simulink library "rewardLibrary"  (R2022b)
settings: Solver=VariableStepAuto  StartTime=0.0  StopTime=10.0  RelTol=1e-3
values from neighbouring files (symbols this model uses):
  accel_vec = (-4:0.5:4)'    [setUpModel.m]
  Ts = 0.1    [setUpMPC.m]
  TsRL = Ts    [setUpRLEnv.m]
  vel_vec = 0:2:20    [setUpModel.m]
undefined symbols (not defined in the file or in its folder): A, B, C, curvature1, D, D_default, DiscIntNeverNeededParam, E, F, gradbp1, k_sigmoid, steer_lim, t_gap, v_set, x_colpen, y_colpen, Z_colpen
libraries: simulink x379, $bdroot x2, mpcadaslib x1
(part 3 of 9)

== system rewardLibrary/Obs // Reward 8-9 ==
  xgap : Inport
  ygap : Inport  Port=2
  v_lead : Inport  Port=3
  v_ego : Inport  Port=4
  v_ref : Inport  Port=5
  e1 : Inport  Port=6
  e2 : Inport  Port=7
  e1dot : Inport  Port=8
  e2dot : Inport  Port=9
  accel : Inport  Port=10
  steer : Inport  Port=11
  collided : Inport  Port=12
  A : Gain  Gain=0
  Abs : Abs  SaturateOnIntegerOverflow=off
  B : Gain  Gain=2000
  Compare To Constant : simulink/Logic and Bit Operations/Compare To Constant  relop=<=  const=6  OutDataTypeStr=boolean
  E : Gain  Gain=2000
  Gain1 : Gain  Gain=20
  Logical Operator1 : Logic  Operator=OR  Inputs=3  AllPortsSameDT=off  OutDataTypeStr=boolean
  Overtaking : Subsystem
  Path following : Subsystem
  Subsystem : Subsystem
  Subsystem2 : Subsystem
  Sum : Sum  Inputs=--+++++
  Zone collision penalty : Lookup_n-D  BreakpointsForDimension1=y_colpen  BreakpointsForDimension2=x_colpen  Table=Z_colpen  ExtrapMethod=Clip  InternalRulePriority=Speed  RndMeth=Simplest
      settings: InputPortMap=u0,u1
      mask Display:
      | image("LookupTable.PNG")
      | port_label('input', 1, 'y')
      | port_label('input', 2, 'x')
      | port_label('output', 1, 'p_col')
  obs : Outport  VectorParamsAs1DForOutWhenUnconnected=off
  Reward : Outport  Port=2  VectorParamsAs1DForOutWhenUnconnected=off
  isDone : Outport  Port=3  VectorParamsAs1DForOutWhenUnconnected=off
  tag scope: onTrack=global, p_col=global
  wires:
  Zone collision penalty/1 -> [p_col], Sum/7
  E/1 -> Sum/2
  Subsystem2/2(failCollided) -> Logical Operator1/2, E/1
  Overtaking/1(r_ot) -> Sum/6
  B/1 -> Sum/4
  Subsystem2/4(overtakeSuccess) -> B/1
  [ry2] -> Overtaking/1(ry)
  Path following/1(r_pf) -> Sum/5
  e2dot/1 -> Subsystem/6(e2dot)
  e1/1 -> Abs/1, Path following/2(e1), Subsystem/3(e1), Subsystem2/2(e1)
  e2/1 -> Subsystem/4(e2), Path following/3(e2), Subsystem2/3(e2)
  v_lead/1 -> Subsystem/7(v_lead)
  xgap/1 -> Subsystem/8(xgap), Subsystem2/4(xgap), Zone collision penalty/2, Overtaking/2(G)
  Subsystem/1(obs) -> obs/1
  e1dot/1 -> Subsystem/5(e1dot)
  Sum/1 -> Reward/1
  Gain1/1 -> Sum/1
  Abs/1 -> Compare To Constant/1
  Compare To Constant/1 -> [onTrack]
  collided/1 -> Subsystem2/5(collided)
  v_ref/1 -> Subsystem/2(v_ref)
  ygap/1 -> Subsystem/9(ygap), Zone collision penalty/1
  Subsystem/2(v_err) -> Path following/1(v_err)
  steer/1 -> Path following/4(steer)
  accel/1 -> Path following/5(accel)
  Logical Operator1/1 -> isDone/1
  v_ego/1 -> Subsystem2/1(v_ego), Subsystem/1(v_ego)
  Subsystem2/1(fail) -> Logical Operator1/1, Gain1/1
  Subsystem2/3(completeCourse) -> A/1, Logical Operator1/3
  A/1 -> Sum/3

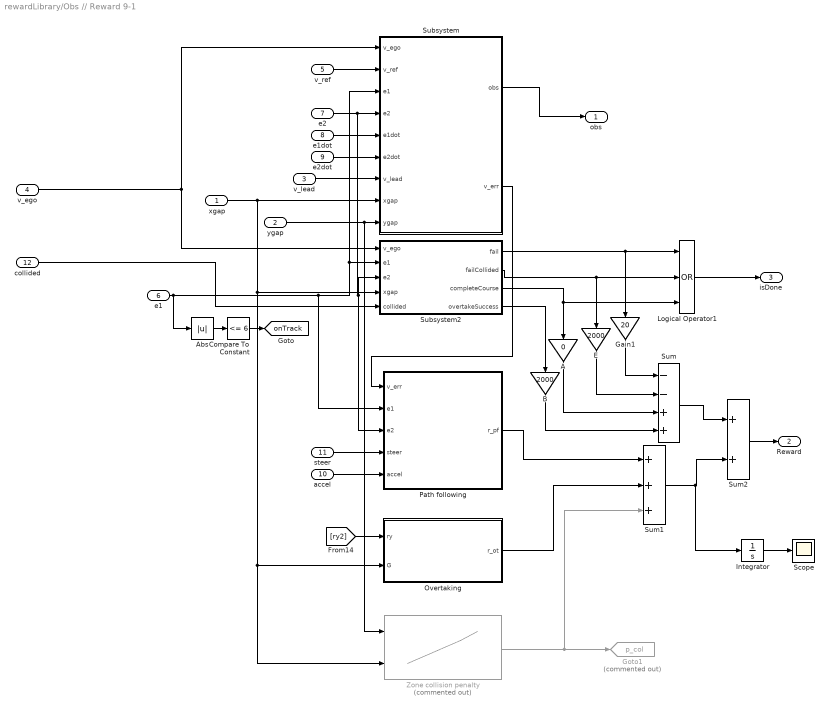
== system rewardLibrary/Obs // Reward 9-1 ==
  xgap : Inport
  ygap : Inport  Port=2
  v_lead : Inport  Port=3
  v_ego : Inport  Port=4
  v_ref : Inport  Port=5
  e1 : Inport  Port=6
  e2 : Inport  Port=7
  e1dot : Inport  Port=8
  e2dot : Inport  Port=9
  accel : Inport  Port=10
  steer : Inport  Port=11
  collided : Inport  Port=12
  A : Gain  Gain=0
  Abs : Abs  SaturateOnIntegerOverflow=off
  B : Gain  Gain=2000
  Compare To Constant : simulink/Logic and Bit Operations/Compare To Constant  relop=<=  const=6  OutDataTypeStr=boolean
  E : Gain  Gain=2000
  Gain1 : Gain  Gain=20
  Goto1 : Goto  Commented=on  GotoTag=p_col  TagVisibility=global
  Integrator : Integrator
  Logical Operator1 : Logic  Operator=OR  Inputs=3  AllPortsSameDT=off  OutDataTypeStr=boolean
  Overtaking : Subsystem
  Path following : Subsystem
  Scope : Scope
  Subsystem : Subsystem
  Subsystem2 : Subsystem
  Sum : Sum  Inputs=--++
  Sum1 : Sum  Inputs=+++
  Sum2 : Sum
  Zone collision penalty : Lookup_n-D  Commented=on  BreakpointsForDimension1=y_colpen  BreakpointsForDimension2=x_colpen  Table=Z_colpen  ExtrapMethod=Clip  InternalRulePriority=Speed  RndMeth=Simplest
      settings: InputPortMap=u0,u1
      mask Display:
      | image("LookupTable.PNG")
      | port_label('input', 1, 'y')
      | port_label('input', 2, 'x')
      | port_label('output', 1, 'p_col')
  obs : Outport  VectorParamsAs1DForOutWhenUnconnected=off
  Reward : Outport  Port=2  VectorParamsAs1DForOutWhenUnconnected=off
  isDone : Outport  Port=3  VectorParamsAs1DForOutWhenUnconnected=off
  tag scope: onTrack=global
  wires:
  Zone collision penalty/1 -> Sum1/3, Goto1/1
  E/1 -> Sum/2
  Subsystem2/2(failCollided) -> Logical Operator1/2, E/1
  Overtaking/1(r_ot) -> Sum1/2
  B/1 -> Sum/4
  Subsystem2/4(overtakeSuccess) -> B/1
  [ry2] -> Overtaking/1(ry)
  Path following/1(r_pf) -> Sum1/1
  e2dot/1 -> Subsystem/6(e2dot)
  e1/1 -> Abs/1, Path following/2(e1), Subsystem/3(e1), Subsystem2/2(e1)
  e2/1 -> Subsystem/4(e2), Path following/3(e2), Subsystem2/3(e2)
  v_lead/1 -> Subsystem/7(v_lead)
  xgap/1 -> Subsystem/8(xgap), Subsystem2/4(xgap), Zone collision penalty/2, Overtaking/2(G)
  Subsystem/1(obs) -> obs/1
  e1dot/1 -> Subsystem/5(e1dot)
  Gain1/1 -> Sum/1
  Abs/1 -> Compare To Constant/1
  Compare To Constant/1 -> [onTrack]
  collided/1 -> Subsystem2/5(collided)
  v_ref/1 -> Subsystem/2(v_ref)
  ygap/1 -> Subsystem/9(ygap), Zone collision penalty/1
  Subsystem/2(v_err) -> Path following/1(v_err)
  steer/1 -> Path following/4(steer)
  accel/1 -> Path following/5(accel)
  Logical Operator1/1 -> isDone/1
  v_ego/1 -> Subsystem2/1(v_ego), Subsystem/1(v_ego)
  Subsystem2/1(fail) -> Logical Operator1/1, Gain1/1
  Subsystem2/3(completeCourse) -> A/1, Logical Operator1/3
  A/1 -> Sum/3
  Sum2/1 -> Reward/1
  Sum/1 -> Sum2/1
  Sum1/1 -> Integrator/1, Sum2/2
  Integrator/1 -> Scope/1

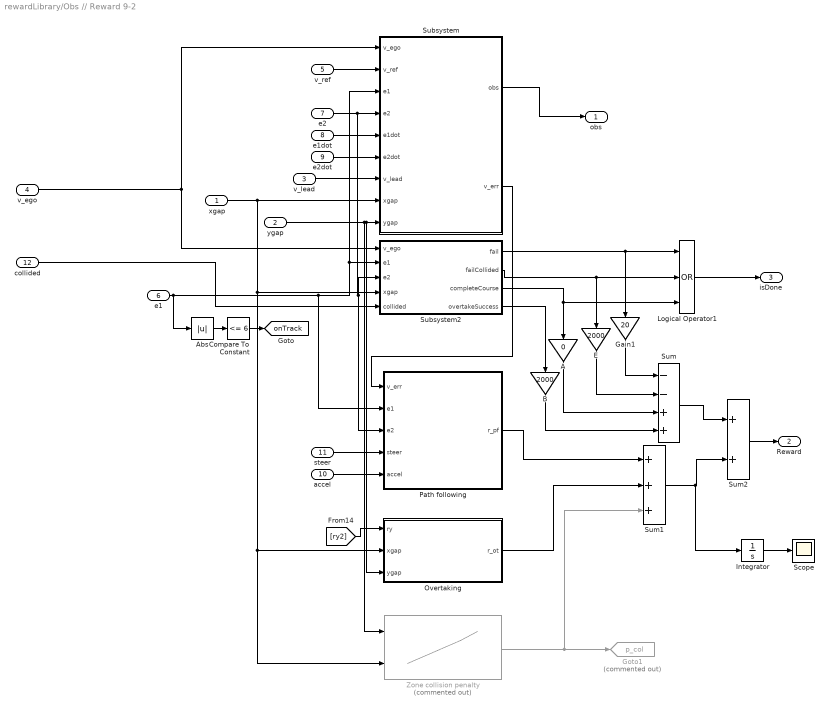
== system rewardLibrary/Obs // Reward 9-2 ==
  xgap : Inport
  ygap : Inport  Port=2
  v_lead : Inport  Port=3
  v_ego : Inport  Port=4
  v_ref : Inport  Port=5
  e1 : Inport  Port=6
  e2 : Inport  Port=7
  e1dot : Inport  Port=8
  e2dot : Inport  Port=9
  accel : Inport  Port=10
  steer : Inport  Port=11
  collided : Inport  Port=12
  A : Gain  Gain=0
  Abs : Abs  SaturateOnIntegerOverflow=off
  B : Gain  Gain=2000
  Compare To Constant : simulink/Logic and Bit Operations/Compare To Constant  relop=<=  const=6  OutDataTypeStr=boolean
  E : Gain  Gain=2000
  Gain1 : Gain  Gain=20
  Goto1 : Goto  Commented=on  GotoTag=p_col  TagVisibility=global
  Integrator : Integrator
  Logical Operator1 : Logic  Operator=OR  Inputs=3  AllPortsSameDT=off  OutDataTypeStr=boolean
  Overtaking : Subsystem
  Path following : Subsystem
  Scope : Scope
  Subsystem : Subsystem
  Subsystem2 : Subsystem
  Sum : Sum  Inputs=--++
  Sum1 : Sum  Inputs=+++
  Sum2 : Sum
  Zone collision penalty : Lookup_n-D  Commented=on  BreakpointsForDimension1=y_colpen  BreakpointsForDimension2=x_colpen  Table=Z_colpen  ExtrapMethod=Clip  InternalRulePriority=Speed  RndMeth=Simplest
      settings: InputPortMap=u0,u1
      mask Display:
      | image("LookupTable.PNG")
      | port_label('input', 1, 'y')
      | port_label('input', 2, 'x')
      | port_label('output', 1, 'p_col')
  obs : Outport  VectorParamsAs1DForOutWhenUnconnected=off
  Reward : Outport  Port=2  VectorParamsAs1DForOutWhenUnconnected=off
  isDone : Outport  Port=3  VectorParamsAs1DForOutWhenUnconnected=off
  tag scope: onTrack=global
  wires:
  Zone collision penalty/1 -> Sum1/3, Goto1/1
  E/1 -> Sum/2
  Subsystem2/2(failCollided) -> Logical Operator1/2, E/1
  Overtaking/1(r_ot) -> Sum1/2
  B/1 -> Sum/4
  Subsystem2/4(overtakeSuccess) -> B/1
  [ry2] -> Overtaking/1(ry)
  Path following/1(r_pf) -> Sum1/1
  e2dot/1 -> Subsystem/6(e2dot)
  e1/1 -> Abs/1, Path following/2(e1), Subsystem/3(e1), Subsystem2/2(e1)
  e2/1 -> Subsystem/4(e2), Path following/3(e2), Subsystem2/3(e2)
  v_lead/1 -> Subsystem/7(v_lead)
  xgap/1 -> Subsystem/8(xgap), Subsystem2/4(xgap), Zone collision penalty/2, Overtaking/2(xgap)
  Subsystem/1(obs) -> obs/1
  e1dot/1 -> Subsystem/5(e1dot)
  Gain1/1 -> Sum/1
  Abs/1 -> Compare To Constant/1
  Compare To Constant/1 -> [onTrack]
  collided/1 -> Subsystem2/5(collided)
  v_ref/1 -> Subsystem/2(v_ref)
  ygap/1 -> Overtaking/3(ygap), Subsystem/9(ygap), Zone collision penalty/1
  Subsystem/2(v_err) -> Path following/1(v_err)
  steer/1 -> Path following/4(steer)
  accel/1 -> Path following/5(accel)
  Logical Operator1/1 -> isDone/1
  v_ego/1 -> Subsystem2/1(v_ego), Subsystem/1(v_ego)
  Subsystem2/1(fail) -> Logical Operator1/1, Gain1/1
  Subsystem2/3(completeCourse) -> A/1, Logical Operator1/3
  A/1 -> Sum/3
  Sum2/1 -> Reward/1
  Sum/1 -> Sum2/1
  Sum1/1 -> Integrator/1, Sum2/2
  Integrator/1 -> Scope/1

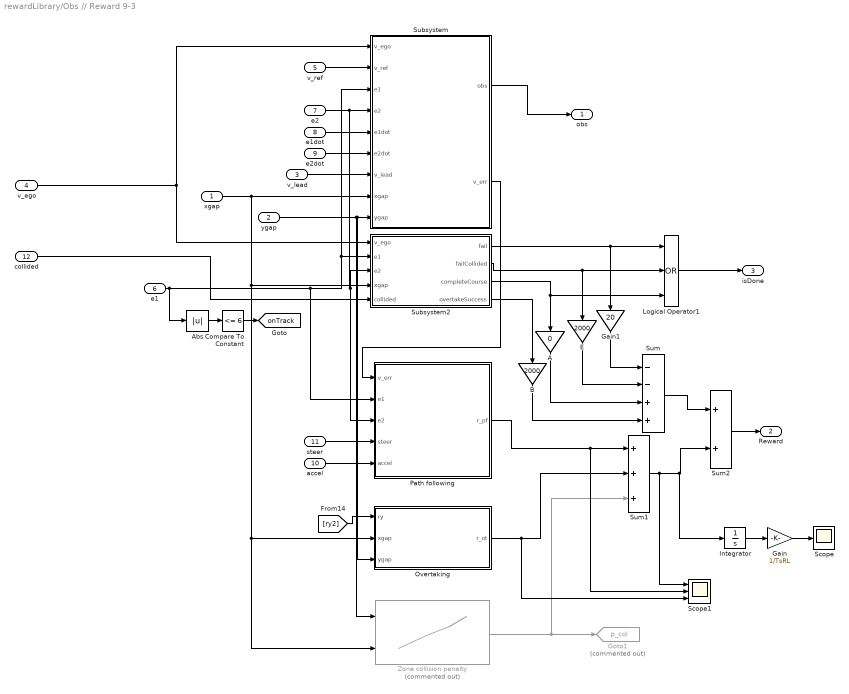
== system rewardLibrary/Obs // Reward 9-3 ==
  xgap : Inport
  ygap : Inport  Port=2
  v_lead : Inport  Port=3
  v_ego : Inport  Port=4
  v_ref : Inport  Port=5
  e1 : Inport  Port=6
  e2 : Inport  Port=7
  e1dot : Inport  Port=8
  e2dot : Inport  Port=9
  accel : Inport  Port=10
  steer : Inport  Port=11
  collided : Inport  Port=12
  A : Gain  Gain=0
  Abs : Abs  SaturateOnIntegerOverflow=off
  B : Gain  Gain=2000
  Compare To Constant : simulink/Logic and Bit Operations/Compare To Constant  relop=<=  const=6  OutDataTypeStr=boolean
  E : Gain  Gain=2000
  Gain : Gain  Gain=1/TsRL
  Gain1 : Gain  Gain=20
  Goto1 : Goto  Commented=on  GotoTag=p_col  TagVisibility=global
  Integrator : Integrator
  Logical Operator1 : Logic  Operator=OR  Inputs=3  AllPortsSameDT=off  OutDataTypeStr=boolean
  Overtaking : Subsystem
  Path following : Subsystem
  Scope : Scope
  Scope1 : Scope  NumInputPorts=3
  Subsystem : Subsystem
  Subsystem2 : Subsystem
  Sum : Sum  Inputs=--++
  Sum1 : Sum  Inputs=+++
  Sum2 : Sum
  Zone collision penalty : Lookup_n-D  Commented=on  BreakpointsForDimension1=y_colpen  BreakpointsForDimension2=x_colpen  Table=Z_colpen  ExtrapMethod=Clip  InternalRulePriority=Speed  RndMeth=Simplest
      settings: InputPortMap=u0,u1
      mask Display:
      | image("LookupTable.PNG")
      | port_label('input', 1, 'y')
      | port_label('input', 2, 'x')
      | port_label('output', 1, 'p_col')
  obs : Outport  VectorParamsAs1DForOutWhenUnconnected=off
  Reward : Outport  Port=2  VectorParamsAs1DForOutWhenUnconnected=off
  isDone : Outport  Port=3  VectorParamsAs1DForOutWhenUnconnected=off
  tag scope: onTrack=global
  wires:
  Zone collision penalty/1 -> Sum1/3, Goto1/1
  E/1 -> Sum/2
  Subsystem2/2(failCollided) -> Logical Operator1/2, E/1
  Overtaking/1(r_ot) -> Scope1/3, Sum1/2
  B/1 -> Sum/4
  Subsystem2/4(overtakeSuccess) -> B/1
  [ry2] -> Overtaking/1(ry)
  Path following/1(r_pf) -> Scope1/2, Sum1/1
  e2dot/1 -> Subsystem/6(e2dot)
  e1/1 -> Abs/1, Path following/2(e1), Subsystem/3(e1), Subsystem2/2(e1)
  e2/1 -> Subsystem/4(e2), Path following/3(e2), Subsystem2/3(e2)
  v_lead/1 -> Subsystem/7(v_lead)
  xgap/1 -> Subsystem/8(xgap), Subsystem2/4(xgap), Zone collision penalty/2, Overtaking/2(xgap)
  Subsystem/1(obs) -> obs/1
  e1dot/1 -> Subsystem/5(e1dot)
  Gain1/1 -> Sum/1
  Abs/1 -> Compare To Constant/1
  Compare To Constant/1 -> [onTrack]
  collided/1 -> Subsystem2/5(collided)
  v_ref/1 -> Subsystem/2(v_ref)
  ygap/1 -> Overtaking/3(ygap), Subsystem/9(ygap), Zone collision penalty/1
  Subsystem/2(v_err) -> Path following/1(v_err)
  steer/1 -> Path following/4(steer)
  accel/1 -> Path following/5(accel)
  Logical Operator1/1 -> isDone/1
  v_ego/1 -> Subsystem2/1(v_ego), Subsystem/1(v_ego)
  Subsystem2/1(fail) -> Logical Operator1/1, Gain1/1
  Subsystem2/3(completeCourse) -> A/1, Logical Operator1/3
  A/1 -> Sum/3
  Sum2/1 -> Reward/1
  Sum/1 -> Sum2/1
  Sum1/1 -> Scope1/1, Integrator/1, Sum2/2
  Gain/1 -> Scope/1
  Integrator/1 -> Gain/1

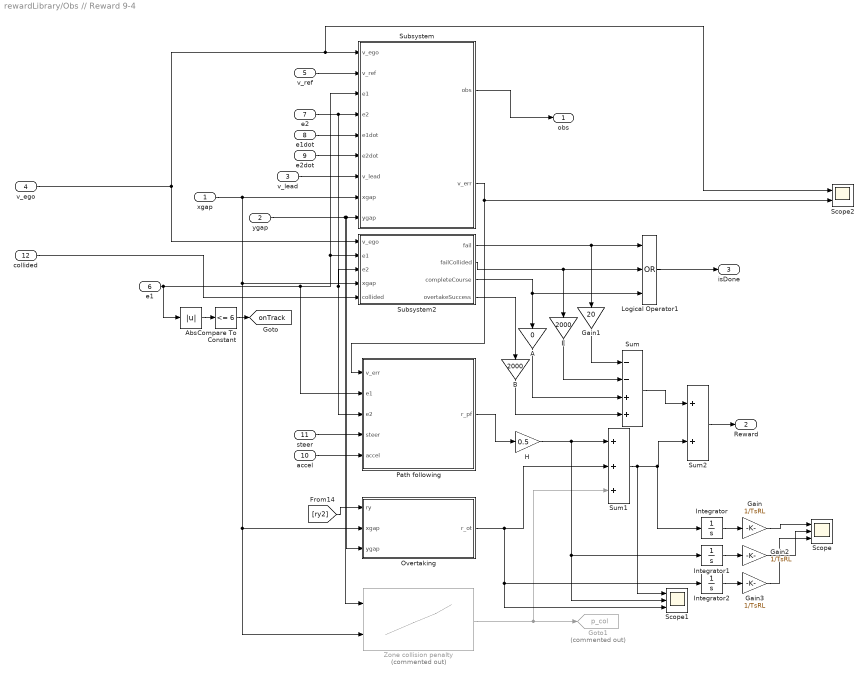
== system rewardLibrary/Obs // Reward 9-4 ==
  xgap : Inport
  ygap : Inport  Port=2
  v_lead : Inport  Port=3
  v_ego : Inport  Port=4
  v_ref : Inport  Port=5
  e1 : Inport  Port=6
  e2 : Inport  Port=7
  e1dot : Inport  Port=8
  e2dot : Inport  Port=9
  accel : Inport  Port=10
  steer : Inport  Port=11
  collided : Inport  Port=12
  A : Gain  Gain=0
  Abs : Abs  SaturateOnIntegerOverflow=off
  B : Gain  Gain=2000
  Compare To Constant : simulink/Logic and Bit Operations/Compare To Constant  relop=<=  const=6  OutDataTypeStr=boolean
  E : Gain  Gain=2000
  Gain : Gain  Gain=1/TsRL
  Gain1 : Gain  Gain=20
  Gain2 : Gain  Gain=1/TsRL
  Gain3 : Gain  Gain=1/TsRL
  Goto1 : Goto  Commented=on  GotoTag=p_col  TagVisibility=global
  H : Gain  Gain=0.5
  Integrator : Integrator
  Integrator1 : Integrator
  Integrator2 : Integrator
  Logical Operator1 : Logic  Operator=OR  Inputs=3  AllPortsSameDT=off  OutDataTypeStr=boolean
  Overtaking : Subsystem
  Path following : Subsystem
  Scope : Scope  NumInputPorts=3
  Scope1 : Scope  NumInputPorts=3
  Scope2 : Scope  NumInputPorts=2
  Subsystem : Subsystem
  Subsystem2 : Subsystem
  Sum : Sum  Inputs=--++
  Sum1 : Sum  Inputs=+++
  Sum2 : Sum
  Zone collision penalty : Lookup_n-D  Commented=on  BreakpointsForDimension1=y_colpen  BreakpointsForDimension2=x_colpen  Table=Z_colpen  ExtrapMethod=Clip  InternalRulePriority=Speed  RndMeth=Simplest
      settings: InputPortMap=u0,u1
      mask Display:
      | image("LookupTable.PNG")
      | port_label('input', 1, 'y')
      | port_label('input', 2, 'x')
      | port_label('output', 1, 'p_col')
  obs : Outport  VectorParamsAs1DForOutWhenUnconnected=off
  Reward : Outport  Port=2  VectorParamsAs1DForOutWhenUnconnected=off
  isDone : Outport  Port=3  VectorParamsAs1DForOutWhenUnconnected=off
  tag scope: onTrack=global
  wires:
  Zone collision penalty/1 -> Sum1/3, Goto1/1
  E/1 -> Sum/2
  Subsystem2/2(failCollided) -> Logical Operator1/2, E/1
  Overtaking/1(r_ot) -> Integrator2/1, Scope1/3, Sum1/2
  B/1 -> Sum/4
  Subsystem2/4(overtakeSuccess) -> B/1
  [ry2] -> Overtaking/1(ry)
  Path following/1(r_pf) -> H/1
  e2dot/1 -> Subsystem/6(e2dot)
  e1/1 -> Abs/1, Path following/2(e1), Subsystem/3(e1), Subsystem2/2(e1)
  e2/1 -> Subsystem/4(e2), Path following/3(e2), Subsystem2/3(e2)
  v_lead/1 -> Subsystem/7(v_lead)
  xgap/1 -> Subsystem/8(xgap), Subsystem2/4(xgap), Zone collision penalty/2, Overtaking/2(xgap)
  Subsystem/1(obs) -> obs/1
  e1dot/1 -> Subsystem/5(e1dot)
  Gain1/1 -> Sum/1
  Abs/1 -> Compare To Constant/1
  Compare To Constant/1 -> [onTrack]
  collided/1 -> Subsystem2/5(collided)
  v_ref/1 -> Subsystem/2(v_ref)
  ygap/1 -> Overtaking/3(ygap), Subsystem/9(ygap), Zone collision penalty/1
  Subsystem/2(v_err) -> Path following/1(v_err), Scope2/2
  steer/1 -> Path following/4(steer)
  accel/1 -> Path following/5(accel)
  Logical Operator1/1 -> isDone/1
  v_ego/1 -> Subsystem2/1(v_ego), Scope2/1, Subsystem/1(v_ego)
  Subsystem2/1(fail) -> Logical Operator1/1, Gain1/1
  Subsystem2/3(completeCourse) -> A/1, Logical Operator1/3
  A/1 -> Sum/3
  Sum2/1 -> Reward/1
  Sum/1 -> Sum2/1
  Sum1/1 -> Scope1/1, Integrator/1, Sum2/2
  Gain/1 -> Scope/1
  Integrator/1 -> Gain/1
  Integrator1/1 -> Gain2/1
  Integrator2/1 -> Gain3/1
  Gain2/1 -> Scope/2
  Gain3/1 -> Scope/3
  H/1 -> Integrator1/1, Scope1/2, Sum1/1

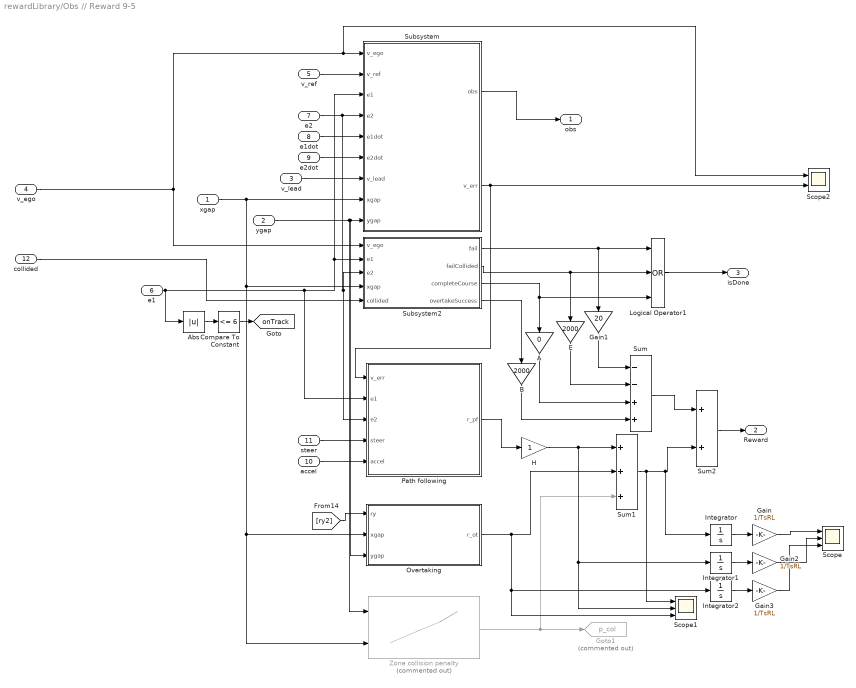
== system rewardLibrary/Obs // Reward 9-5 ==
  xgap : Inport
  ygap : Inport  Port=2
  v_lead : Inport  Port=3
  v_ego : Inport  Port=4
  v_ref : Inport  Port=5
  e1 : Inport  Port=6
  e2 : Inport  Port=7
  e1dot : Inport  Port=8
  e2dot : Inport  Port=9
  accel : Inport  Port=10
  steer : Inport  Port=11
  collided : Inport  Port=12
  A : Gain  Gain=0
  Abs : Abs  SaturateOnIntegerOverflow=off
  B : Gain  Gain=2000
  Compare To Constant : simulink/Logic and Bit Operations/Compare To Constant  relop=<=  const=6  OutDataTypeStr=boolean
  E : Gain  Gain=2000
  Gain : Gain  Gain=1/TsRL
  Gain1 : Gain  Gain=20
  Gain2 : Gain  Gain=1/TsRL
  Gain3 : Gain  Gain=1/TsRL
  Goto1 : Goto  Commented=on  GotoTag=p_col  TagVisibility=global
  H : Gain
  Integrator : Integrator
  Integrator1 : Integrator
  Integrator2 : Integrator
  Logical Operator1 : Logic  Operator=OR  Inputs=3  AllPortsSameDT=off  OutDataTypeStr=boolean
  Overtaking : Subsystem
  Path following : Subsystem
  Scope : Scope  NumInputPorts=3
  Scope1 : Scope  NumInputPorts=3
  Scope2 : Scope  NumInputPorts=2
  Subsystem : Subsystem
  Subsystem2 : Subsystem
  Sum : Sum  Inputs=--++
  Sum1 : Sum  Inputs=+++
  Sum2 : Sum
  Zone collision penalty : Lookup_n-D  Commented=on  BreakpointsForDimension1=y_colpen  BreakpointsForDimension2=x_colpen  Table=Z_colpen  ExtrapMethod=Clip  InternalRulePriority=Speed  RndMeth=Simplest
      settings: InputPortMap=u0,u1
      mask Display:
      | image("LookupTable.PNG")
      | port_label('input', 1, 'y')
      | port_label('input', 2, 'x')
      | port_label('output', 1, 'p_col')
  obs : Outport  VectorParamsAs1DForOutWhenUnconnected=off
  Reward : Outport  Port=2  VectorParamsAs1DForOutWhenUnconnected=off
  isDone : Outport  Port=3  VectorParamsAs1DForOutWhenUnconnected=off
  tag scope: onTrack=global
  wires:
  Zone collision penalty/1 -> Sum1/3, Goto1/1
  E/1 -> Sum/2
  Subsystem2/2(failCollided) -> Logical Operator1/2, E/1
  Overtaking/1(r_ot) -> Integrator2/1, Scope1/3, Sum1/2
  B/1 -> Sum/4
  Subsystem2/4(overtakeSuccess) -> B/1
  [ry2] -> Overtaking/1(ry)
  Path following/1(r_pf) -> H/1
  e2dot/1 -> Subsystem/6(e2dot)
  e1/1 -> Abs/1, Path following/2(e1), Subsystem/3(e1), Subsystem2/2(e1)
  e2/1 -> Subsystem/4(e2), Path following/3(e2), Subsystem2/3(e2)
  v_lead/1 -> Subsystem/7(v_lead)
  xgap/1 -> Subsystem/8(xgap), Subsystem2/4(xgap), Zone collision penalty/2, Overtaking/2(xgap)
  Subsystem/1(obs) -> obs/1
  e1dot/1 -> Subsystem/5(e1dot)
  Gain1/1 -> Sum/1
  Abs/1 -> Compare To Constant/1
  Compare To Constant/1 -> [onTrack]
  collided/1 -> Subsystem2/5(collided)
  v_ref/1 -> Subsystem/2(v_ref)
  ygap/1 -> Overtaking/3(ygap), Subsystem/9(ygap), Zone collision penalty/1
  Subsystem/2(v_err) -> Path following/1(v_err), Scope2/2
  steer/1 -> Path following/4(steer)
  accel/1 -> Path following/5(accel)
  Logical Operator1/1 -> isDone/1
  v_ego/1 -> Subsystem2/1(v_ego), Scope2/1, Subsystem/1(v_ego)
  Subsystem2/1(fail) -> Logical Operator1/1, Gain1/1
  Subsystem2/3(completeCourse) -> A/1, Logical Operator1/3
  A/1 -> Sum/3
  Sum2/1 -> Reward/1
  Sum/1 -> Sum2/1
  Sum1/1 -> Scope1/1, Integrator/1, Sum2/2
  Gain/1 -> Scope/1
  Integrator/1 -> Gain/1
  Integrator1/1 -> Gain2/1
  Integrator2/1 -> Gain3/1
  Gain2/1 -> Scope/2
  Gain3/1 -> Scope/3
  H/1 -> Integrator1/1, Scope1/2, Sum1/1

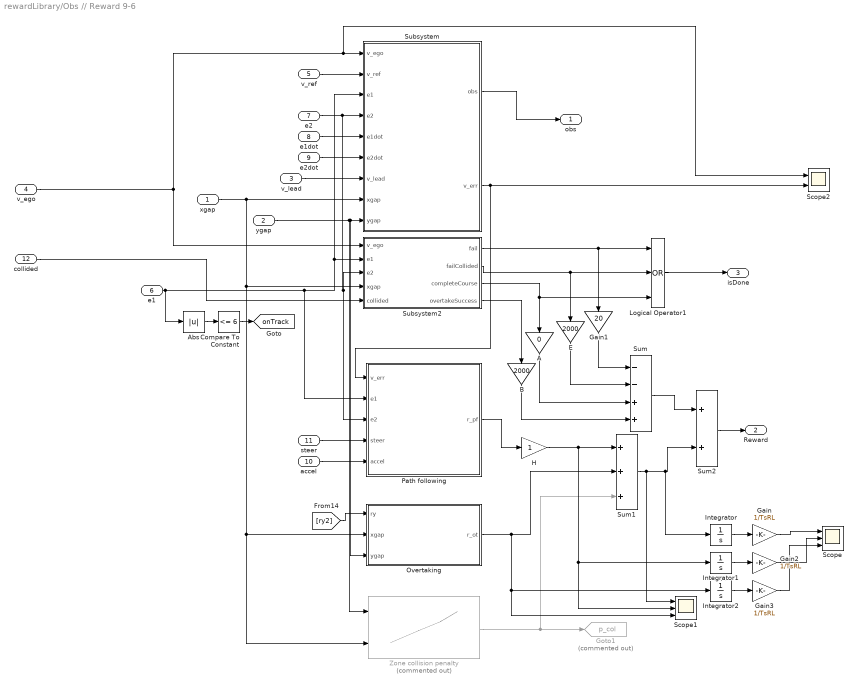
== system rewardLibrary/Obs // Reward 9-6 ==
  xgap : Inport
  ygap : Inport  Port=2
  v_lead : Inport  Port=3
  v_ego : Inport  Port=4
  v_ref : Inport  Port=5
  e1 : Inport  Port=6
  e2 : Inport  Port=7
  e1dot : Inport  Port=8
  e2dot : Inport  Port=9
  accel : Inport  Port=10
  steer : Inport  Port=11
  collided : Inport  Port=12
  A : Gain  Gain=0
  Abs : Abs  SaturateOnIntegerOverflow=off
  B : Gain  Gain=2000
  Compare To Constant : simulink/Logic and Bit Operations/Compare To Constant  relop=<=  const=6  OutDataTypeStr=boolean
  E : Gain  Gain=2000
  Gain : Gain  Gain=1/TsRL
  Gain1 : Gain  Gain=20
  Gain2 : Gain  Gain=1/TsRL
  Gain3 : Gain  Gain=1/TsRL
  Goto1 : Goto  Commented=on  GotoTag=p_col  TagVisibility=global
  H : Gain
  Integrator : Integrator
  Integrator1 : Integrator
  Integrator2 : Integrator
  Logical Operator1 : Logic  Operator=OR  Inputs=3  AllPortsSameDT=off  OutDataTypeStr=boolean
  Overtaking : Subsystem
  Path following : Subsystem
  Scope : Scope  NumInputPorts=3
  Scope1 : Scope  NumInputPorts=3
  Scope2 : Scope  NumInputPorts=2
  Subsystem : Subsystem
  Subsystem2 : Subsystem
  Sum : Sum  Inputs=--++
  Sum1 : Sum  Inputs=+++
  Sum2 : Sum
  Zone collision penalty : Lookup_n-D  Commented=on  BreakpointsForDimension1=y_colpen  BreakpointsForDimension2=x_colpen  Table=Z_colpen  ExtrapMethod=Clip  InternalRulePriority=Speed  RndMeth=Simplest
      settings: InputPortMap=u0,u1
      mask Display:
      | image("LookupTable.PNG")
      | port_label('input', 1, 'y')
      | port_label('input', 2, 'x')
      | port_label('output', 1, 'p_col')
  obs : Outport  VectorParamsAs1DForOutWhenUnconnected=off
  Reward : Outport  Port=2  VectorParamsAs1DForOutWhenUnconnected=off
  isDone : Outport  Port=3  VectorParamsAs1DForOutWhenUnconnected=off
  tag scope: onTrack=global
  wires:
  Zone collision penalty/1 -> Sum1/3, Goto1/1
  E/1 -> Sum/2
  Subsystem2/2(failCollided) -> Logical Operator1/2, E/1
  Overtaking/1(r_ot) -> Integrator2/1, Scope1/3, Sum1/2
  B/1 -> Sum/4
  Subsystem2/4(overtakeSuccess) -> B/1
  [ry2] -> Overtaking/1(ry)
  Path following/1(r_pf) -> H/1
  e2dot/1 -> Subsystem/6(e2dot)
  e1/1 -> Abs/1, Path following/2(e1), Subsystem/3(e1), Subsystem2/2(e1)
  e2/1 -> Subsystem/4(e2), Path following/3(e2), Subsystem2/3(e2)
  v_lead/1 -> Subsystem/7(v_lead)
  xgap/1 -> Subsystem/8(xgap), Subsystem2/4(xgap), Zone collision penalty/2, Overtaking/2(xgap)
  Subsystem/1(obs) -> obs/1
  e1dot/1 -> Subsystem/5(e1dot)
  Gain1/1 -> Sum/1
  Abs/1 -> Compare To Constant/1
  Compare To Constant/1 -> [onTrack]
  collided/1 -> Subsystem2/5(collided)
  v_ref/1 -> Subsystem/2(v_ref)
  ygap/1 -> Overtaking/3(ygap), Subsystem/9(ygap), Zone collision penalty/1
  Subsystem/2(v_err) -> Path following/1(v_err), Scope2/2
  steer/1 -> Path following/4(steer)
  accel/1 -> Path following/5(accel)
  Logical Operator1/1 -> isDone/1
  v_ego/1 -> Subsystem2/1(v_ego), Scope2/1, Subsystem/1(v_ego)
  Subsystem2/1(fail) -> Logical Operator1/1, Gain1/1
  Subsystem2/3(completeCourse) -> A/1, Logical Operator1/3
  A/1 -> Sum/3
  Sum2/1 -> Reward/1
  Sum/1 -> Sum2/1
  Sum1/1 -> Scope1/1, Integrator/1, Sum2/2
  Gain/1 -> Scope/1
  Integrator/1 -> Gain/1
  Integrator1/1 -> Gain2/1
  Integrator2/1 -> Gain3/1
  Gain2/1 -> Scope/2
  Gain3/1 -> Scope/3
  H/1 -> Integrator1/1, Scope1/2, Sum1/1

== system rewardLibrary/Reward 0-0 ==
  d_rel : Inport
  v_lead : Inport  Port=2
  v_ego : Inport  Port=3
  e1 : Inport  Port=4
  e2 : Inport  Port=5
  e1dot : Inport  Port=6
  e2dot : Inport  Port=7
  accel : Inport  Port=8
  steer : Inport  Port=9
  Ft : Gain  Gain=10
  Subsystem : Subsystem
  Subsystem1 : Subsystem
  Subsystem2 : Subsystem
  Sum : Sum  Inputs=-+|
  obs : Outport  VectorParamsAs1DForOutWhenUnconnected=off
  Reward : Outport  Port=2  VectorParamsAs1DForOutWhenUnconnected=off
  isDone : Outport  Port=3  VectorParamsAs1DForOutWhenUnconnected=off
  wires:
  e2dot/1 -> Subsystem/7(e2dot)
  e1/1 -> Subsystem/4(e1), Subsystem1/2(e1), Subsystem2/3(e1)
  e2/1 -> Subsystem/5(e2)
  v_ego/1 -> Subsystem2/2(v_ego), Subsystem/1(v_ego)
  accel/1 -> Subsystem1/4(a)
  Subsystem2/1(isDone) -> Ft/1, isDone/1
  Subsystem/2(v_err) -> Subsystem1/3(ev)
  v_lead/1 -> Subsystem/3(v_lead)
  d_rel/1 -> Subsystem/2(d_rel), Subsystem2/1(d_rel)
  steer/1 -> Subsystem1/1(u)
  Subsystem/1(obs) -> obs/1
  e1dot/1 -> Subsystem/6(e1dot)
  Subsystem1/1(reward) -> Sum/2
  Sum/1 -> Reward/1
  Ft/1 -> Sum/1

== system rewardLibrary/Reward 1-1 ==
  xgap : Inport
  ygap : Inport  Port=2
  v_lead : Inport  Port=3
  v_ego : Inport  Port=4
  v_ref : Inport  Port=5
  e1 : Inport  Port=6
  e2 : Inport  Port=7
  e1dot : Inport  Port=8
  e2dot : Inport  Port=9
  accel : Inport  Port=10
  steer : Inport  Port=11
  collided : Inport  Port=12
  Abs : Abs  SaturateOnIntegerOverflow=off
  Compare To Constant : simulink/Logic and Bit Operations/Compare To Constant  relop=<=  const=6  OutDataTypeStr=boolean
  Gain : Gain  Gain=10
  Subsystem : Subsystem
  Subsystem1 : Subsystem
  Subsystem2 : Subsystem
  Sum : Sum  Inputs=-+|
  Terminator{,1..3} (4 alike) : Terminator
  obs : Outport  VectorParamsAs1DForOutWhenUnconnected=off
  Reward : Outport  Port=2  VectorParamsAs1DForOutWhenUnconnected=off
  isDone : Outport  Port=3  VectorParamsAs1DForOutWhenUnconnected=off
  tag scope: onTrack=global
  wires:
  e2dot/1 -> Subsystem/6(e2dot)
  e1/1 -> Abs/1, Subsystem/3(e1), Subsystem2/2(e1), Subsystem1/2(e1)
  e2/1 -> Subsystem/4(e2)
  v_ego/1 -> Subsystem2/1(v_ego), Subsystem/1(v_ego)
  Subsystem2/1(isDone) -> Gain/1, isDone/1
  Subsystem/2(v_err) -> Subsystem1/3(v_err)
  v_lead/1 -> Terminator/1
  xgap/1 -> Terminator1/1
  steer/1 -> Subsystem1/1(steer)
  Subsystem/1(obs) -> obs/1
  e1dot/1 -> Subsystem/5(e1dot)
  Subsystem1/1(reward) -> Sum/2
  Sum/1 -> Reward/1
  Gain/1 -> Sum/1
  Abs/1 -> Compare To Constant/1
  Compare To Constant/1 -> [onTrack]
  collided/1 -> Terminator3/1
  v_ref/1 -> Subsystem/2(v_ref)
  ygap/1 -> Terminator2/1
  accel/1 -> Subsystem1/4(accel)

== system rewardLibrary/MPC Based Controller/Pedal map ==
  vx : Inport
  a : Inport  Port=2
  Dead Zone1 : DeadZone  LowerValue=-0.001  UpperValue=0.001
  Dead Zone2 : DeadZone  LowerValue=-0.001  UpperValue=0.001
  Gain : Gain  Gain=-1
  Pedal map : Lookup_n-D  BreakpointsForDimension1=vel_vec  BreakpointsForDimension2=accel_vec  Table=pedal_map'  InternalRulePriority=Speed  RndMeth=Simplest
      settings: InputPortMap=u0,u1
  Saturation : Saturate  UpperLimit=1  LowerLimit=0
  Saturation1 : Saturate  UpperLimit=0  LowerLimit=-1
  Out1 : Outport
  Out2 : Outport  Port=2
  wires:
  a/1 -> Pedal map/2
  Dead Zone2/1 -> Out2/1
  Dead Zone1/1 -> Out1/1
  vx/1 -> Pedal map/1
  Gain/1 -> Dead Zone2/1
  Saturation1/1 -> Gain/1
  Saturation/1 -> Dead Zone1/1
  Pedal map/1 -> Saturation1/1, Saturation/1

== system rewardLibrary/MPC Based Controller/Sensor Dynamics ==
  Current curvature : Inport
  Longitudinal velocity : Inport  Port=2
  Lateral velocity : Inport  Port=3
  Yaw rate : Inport  Port=4
  Integrator : Integrator
  Integrator2 : Integrator
  Mux1 : Mux  Inputs=[1 1 1]
  Product : Product
  Subtract : Sum  Inputs=-+
  e1dot : Fcn  Expr=u(1)*u(3)+u(2)
  Lateral deviation : Outport  VectorParamsAs1DForOutWhenUnconnected=off
  Relative yaw angle : Outport  Port=2  VectorParamsAs1DForOutWhenUnconnected=off
  wires:
  Current curvature/1 -> Product/2
  Integrator2/1 -> Mux1/3, Relative yaw angle/1  "e2"
  Mux1/1 -> e1dot/1
  e1dot/1 -> Integrator/1
  Longitudinal velocity/1 -> Product/1, Mux1/1
  Lateral velocity/1 -> Mux1/2
  Integrator/1 -> Lateral deviation/1  "e1"
  Product/1 -> Subtract/1
  Yaw rate/1 -> Subtract/2
  Subtract/1 -> Integrator2/1  "e2dot"

== system rewardLibrary/Obs // Reward 1-2/Subsystem ==
  v_ego : Inport
  v_ref : Inport  Port=2
  e1 : Inport  Port=3
  e2 : Inport  Port=4
  e1dot : Inport  Port=5
  e2dot : Inport  Port=6
  Add : Sum  Inputs=+-
  Discrete-Time Integrator1 : DiscreteIntegrator  SampleTime=-1  ICPrevOutput=DiscIntNeverNeededParam  ICPrevScaledInput=DiscIntNeverNeededParam
  Discrete-Time Integrator2 : DiscreteIntegrator  SampleTime=-1  ICPrevOutput=DiscIntNeverNeededParam  ICPrevScaledInput=DiscIntNeverNeededParam
  Discrete-Time Integrator3 : DiscreteIntegrator  SampleTime=-1  ICPrevOutput=DiscIntNeverNeededParam  ICPrevScaledInput=DiscIntNeverNeededParam
  Lateral deviation : Scope
  Mux : Mux  Inputs=9
  obs : Outport  VectorParamsAs1DForOutWhenUnconnected=off
  v_err : Outport  Port=2  VectorParamsAs1DForOutWhenUnconnected=off
  wires:
  Add/1 -> v_err/1, Mux/2, Discrete-Time Integrator1/1
  Discrete-Time Integrator3/1 -> Mux/6  "integral_error"
  v_ego/1 -> Add/2, Mux/3
  e1/1 -> Lateral deviation/1, Mux/5, Discrete-Time Integrator2/1
  Discrete-Time Integrator1/1 -> Mux/1  "integral_error"
  e2/1 -> Mux/7, Discrete-Time Integrator3/1
  Discrete-Time Integrator2/1 -> Mux/4  "integral_error"
  Mux/1 -> obs/1
  e1dot/1 -> Mux/8
  e2dot/1 -> Mux/9
  v_ref/1 -> Add/1  "d_rel"

== system rewardLibrary/Obs // Reward 1-2/Subsystem1 ==
  steer : Inport
  e1 : Inport  Port=2
  v_err : Inport  Port=3
  accel : Inport  Port=4
  Compare To Constant1 : simulink/Logic and Bit Operations/Compare To Constant  relop=<  const=0.25  OutDataTypeStr=boolean
  Gain : Gain  Gain=100
  Gain1 : Gain  Gain=0
  Gain2 : Gain  Gain=200
  Gain3 : Gain  Gain=2
  Gain4 : Gain  Gain=1e-3
  Gain7 : Gain  Gain=10
  Square{,1..2,5} (4 alike) : Math  Operator=square  SignedPower=on
  Sum : Sum  Inputs=----
  Sum1 : Sum
  Unit Delay : UnitDelay  SampleTime=-1  HasFrameUpgradeWarning=on
  Unit Delay1 : UnitDelay  SampleTime=-1  HasFrameUpgradeWarning=on
  reward : Outport  VectorParamsAs1DForOutWhenUnconnected=off
  wires:
  e1/1 -> Square/1
  Gain/1 -> Sum/1
  Square/1 -> Compare To Constant1/1, Gain/1
  steer/1 -> Unit Delay/1
  Square2/1 -> Gain2/1
  Unit Delay/1 -> Square2/1
  Square5/1 -> Gain7/1
  Gain7/1 -> Sum/3
  v_err/1 -> Square5/1
  Gain2/1 -> Sum/2
  Sum1/1 -> reward/1
  Compare To Constant1/1 -> Gain3/1
  Gain3/1 -> Sum1/1
  Sum/1 -> Gain4/1
  Gain4/1 -> Sum1/2
  accel/1 -> Unit Delay1/1
  Unit Delay1/1 -> Square1/1
  Square1/1 -> Gain1/1
  Gain1/1 -> Sum/4

== system rewardLibrary/Obs // Reward 1-2/Subsystem2 ==
  v_ego : Inport
  e1 : Inport  Port=2
  e2 : Inport  Port=3
  AND : Logic  IconShape=distinctive  AllPortsSameDT=off  OutDataTypeStr=boolean
  Abs : Abs  SaturateOnIntegerOverflow=off
  Abs1 : Abs  SaturateOnIntegerOverflow=off
  Lateral deviation : simulink/Logic and Bit Operations/Compare To Constant  relop=>  const=8  OutDataTypeStr=boolean
  Logical Operator : Logic  Operator=OR  Inputs=3  AllPortsSameDT=off  OutDataTypeStr=boolean
  R2D : Gain  Gain=180/pi
  Relative yaw angle : simulink/Logic and Bit Operations/Compare To Constant  relop=>  const=60  OutDataTypeStr=boolean
  Velocity : simulink/Logic and Bit Operations/Compare To Constant  relop=<  const=0.5  OutDataTypeStr=boolean
  Velocity1 : simulink/Logic and Bit Operations/Compare To Constant  relop=<  const=10  OutDataTypeStr=boolean
  isDone : Outport  VectorParamsAs1DForOutWhenUnconnected=off
  wires:
  Velocity/1 -> Logical Operator/1
  Logical Operator/1 -> isDone/1
  v_ego/1 -> Velocity1/1, Velocity/1
  Abs/1 -> Lateral deviation/1
  Lateral deviation/1 -> Logical Operator/2
  e1/1 -> Abs/1
  Velocity1/1 -> AND/1
  e2/1 -> Abs1/1
  Abs1/1 -> R2D/1
  R2D/1 -> Relative yaw angle/1
  Relative yaw angle/1 -> AND/2
  AND/1 -> Logical Operator/3

== system rewardLibrary/Obs // Reward 1-3/Subsystem ==
  v_ego : Inport
  v_ref : Inport  Port=2
  e1 : Inport  Port=3
  e2 : Inport  Port=4
  e1dot : Inport  Port=5
  e2dot : Inport  Port=6
  Add : Sum  Inputs=+-
  Discrete-Time Integrator1 : DiscreteIntegrator  SampleTime=-1  ICPrevOutput=DiscIntNeverNeededParam  ICPrevScaledInput=DiscIntNeverNeededParam
  Discrete-Time Integrator2 : DiscreteIntegrator  SampleTime=-1  ICPrevOutput=DiscIntNeverNeededParam  ICPrevScaledInput=DiscIntNeverNeededParam
  Discrete-Time Integrator3 : DiscreteIntegrator  SampleTime=-1  ICPrevOutput=DiscIntNeverNeededParam  ICPrevScaledInput=DiscIntNeverNeededParam
  Lateral deviation : Scope
  Mux : Mux  Inputs=9
  obs : Outport  VectorParamsAs1DForOutWhenUnconnected=off
  v_err : Outport  Port=2  VectorParamsAs1DForOutWhenUnconnected=off
  wires:
  Add/1 -> v_err/1, Mux/2, Discrete-Time Integrator1/1
  Discrete-Time Integrator3/1 -> Mux/6  "integral_error"
  v_ego/1 -> Add/2, Mux/3
  e1/1 -> Lateral deviation/1, Mux/5, Discrete-Time Integrator2/1
  Discrete-Time Integrator1/1 -> Mux/1  "integral_error"
  e2/1 -> Mux/7, Discrete-Time Integrator3/1
  Discrete-Time Integrator2/1 -> Mux/4  "integral_error"
  Mux/1 -> obs/1
  e1dot/1 -> Mux/8
  e2dot/1 -> Mux/9
  v_ref/1 -> Add/1  "d_rel"

== system rewardLibrary/Obs // Reward 1-3/Subsystem1 ==
  steer : Inport
  e1 : Inport  Port=2
  v_err : Inport  Port=3
  accel : Inport  Port=4
  Compare To Constant1 : simulink/Logic and Bit Operations/Compare To Constant  relop=<  const=0.25  OutDataTypeStr=boolean
  Gain : Gain  Gain=100
  Gain1 : Gain  Gain=0
  Gain2 : Gain  Gain=200
  Gain3 : Gain  Gain=2
  Gain4 : Gain  Gain=1e-3
  Gain7 : Gain  Gain=10
  Square{,1..2,5} (4 alike) : Math  Operator=square  SignedPower=on
  Sum : Sum  Inputs=----
  Sum1 : Sum
  Unit Delay : UnitDelay  SampleTime=-1  HasFrameUpgradeWarning=on
  Unit Delay1 : UnitDelay  SampleTime=-1  HasFrameUpgradeWarning=on
  reward : Outport  VectorParamsAs1DForOutWhenUnconnected=off
  wires:
  e1/1 -> Square/1
  Gain/1 -> Sum/1
  Square/1 -> Compare To Constant1/1, Gain/1
  steer/1 -> Unit Delay/1
  Square2/1 -> Gain2/1
  Unit Delay/1 -> Square2/1
  Square5/1 -> Gain7/1
  Gain7/1 -> Sum/3
  v_err/1 -> Square5/1
  Gain2/1 -> Sum/2
  Sum1/1 -> reward/1
  Compare To Constant1/1 -> Gain3/1
  Gain3/1 -> Sum1/1
  Sum/1 -> Gain4/1
  Gain4/1 -> Sum1/2
  accel/1 -> Unit Delay1/1
  Unit Delay1/1 -> Square1/1
  Square1/1 -> Gain1/1
  Gain1/1 -> Sum/4

== system rewardLibrary/Obs // Reward 1-3/Subsystem2 ==
  v_ego : Inport
  e1 : Inport  Port=2
  e2 : Inport  Port=3
  AND : Logic  IconShape=distinctive  AllPortsSameDT=off  OutDataTypeStr=boolean
  Abs : Abs  SaturateOnIntegerOverflow=off
  Abs1 : Abs  SaturateOnIntegerOverflow=off
  Lateral deviation : simulink/Logic and Bit Operations/Compare To Constant  relop=>  const=8  OutDataTypeStr=boolean
  Logical Operator : Logic  Operator=OR  Inputs=3  AllPortsSameDT=off  OutDataTypeStr=boolean
  R2D : Gain  Gain=180/pi
  Relative yaw angle : simulink/Logic and Bit Operations/Compare To Constant  relop=>  const=60  OutDataTypeStr=boolean
  Velocity : simulink/Logic and Bit Operations/Compare To Constant  relop=<  const=0.5  OutDataTypeStr=boolean
  Velocity1 : simulink/Logic and Bit Operations/Compare To Constant  relop=<  const=10  OutDataTypeStr=boolean
  isDone : Outport  VectorParamsAs1DForOutWhenUnconnected=off
  wires:
  Velocity/1 -> Logical Operator/1
  Logical Operator/1 -> isDone/1
  v_ego/1 -> Velocity1/1, Velocity/1
  Abs/1 -> Lateral deviation/1
  Lateral deviation/1 -> Logical Operator/2
  e1/1 -> Abs/1
  Velocity1/1 -> AND/1
  e2/1 -> Abs1/1
  Abs1/1 -> R2D/1
  R2D/1 -> Relative yaw angle/1
  Relative yaw angle/1 -> AND/2
  AND/1 -> Logical Operator/3

== system rewardLibrary/Obs // Reward 1-4/Subsystem ==
  v_ego : Inport
  v_ref : Inport  Port=2
  e1 : Inport  Port=3
  e2 : Inport  Port=4
  e1dot : Inport  Port=5
  e2dot : Inport  Port=6
  Add : Sum  Inputs=+-
  Discrete-Time Integrator1 : DiscreteIntegrator  SampleTime=-1  ICPrevOutput=DiscIntNeverNeededParam  ICPrevScaledInput=DiscIntNeverNeededParam
  Discrete-Time Integrator2 : DiscreteIntegrator  SampleTime=-1  ICPrevOutput=DiscIntNeverNeededParam  ICPrevScaledInput=DiscIntNeverNeededParam
  Discrete-Time Integrator3 : DiscreteIntegrator  SampleTime=-1  ICPrevOutput=DiscIntNeverNeededParam  ICPrevScaledInput=DiscIntNeverNeededParam
  Lateral deviation : Scope
  Mux : Mux  Inputs=9
  obs : Outport  VectorParamsAs1DForOutWhenUnconnected=off
  v_err : Outport  Port=2  VectorParamsAs1DForOutWhenUnconnected=off
  wires:
  Add/1 -> v_err/1, Mux/2, Discrete-Time Integrator1/1
  Discrete-Time Integrator3/1 -> Mux/6  "integral_error"
  v_ego/1 -> Add/2, Mux/3
  e1/1 -> Lateral deviation/1, Mux/5, Discrete-Time Integrator2/1
  Discrete-Time Integrator1/1 -> Mux/1  "integral_error"
  e2/1 -> Mux/7, Discrete-Time Integrator3/1
  Discrete-Time Integrator2/1 -> Mux/4  "integral_error"
  Mux/1 -> obs/1
  e1dot/1 -> Mux/8
  e2dot/1 -> Mux/9
  v_ref/1 -> Add/1  "d_rel"

== system rewardLibrary/Obs // Reward 1-4/Subsystem1 ==
  steer : Inport
  e1 : Inport  Port=2
  v_err : Inport  Port=3
  accel : Inport  Port=4
  Compare To Constant1 : simulink/Logic and Bit Operations/Compare To Constant  relop=<  const=0.25  OutDataTypeStr=boolean
  Gain : Gain  Gain=100
  Gain1 : Gain  Gain=0
  Gain2 : Gain  Gain=500
  Gain3 : Gain  Gain=2
  Gain4 : Gain  Gain=1e-3
  Gain7 : Gain  Gain=10
  Square{,1..2,5} (4 alike) : Math  Operator=square  SignedPower=on
  Sum : Sum  Inputs=----
  Sum1 : Sum
  Unit Delay : UnitDelay  SampleTime=-1  HasFrameUpgradeWarning=on
  Unit Delay1 : UnitDelay  SampleTime=-1  HasFrameUpgradeWarning=on
  reward : Outport  VectorParamsAs1DForOutWhenUnconnected=off
  wires:
  e1/1 -> Square/1
  Gain/1 -> Sum/1
  Square/1 -> Compare To Constant1/1, Gain/1
  steer/1 -> Unit Delay/1
  Square2/1 -> Gain2/1
  Unit Delay/1 -> Square2/1
  Square5/1 -> Gain7/1
  Gain7/1 -> Sum/3
  v_err/1 -> Square5/1
  Gain2/1 -> Sum/2
  Sum1/1 -> reward/1
  Compare To Constant1/1 -> Gain3/1
  Gain3/1 -> Sum1/1
  Sum/1 -> Gain4/1
  Gain4/1 -> Sum1/2
  accel/1 -> Unit Delay1/1
  Unit Delay1/1 -> Square1/1
  Square1/1 -> Gain1/1
  Gain1/1 -> Sum/4

== system rewardLibrary/Obs // Reward 1-4/Subsystem2 ==
  v_ego : Inport
  e1 : Inport  Port=2
  e2 : Inport  Port=3
  AND : Logic  IconShape=distinctive  AllPortsSameDT=off  OutDataTypeStr=boolean
  Abs : Abs  SaturateOnIntegerOverflow=off
  Abs1 : Abs  SaturateOnIntegerOverflow=off
  Lateral deviation : simulink/Logic and Bit Operations/Compare To Constant  relop=>  const=8  OutDataTypeStr=boolean
  Logical Operator : Logic  Operator=OR  Inputs=3  AllPortsSameDT=off  OutDataTypeStr=boolean
  R2D : Gain  Gain=180/pi
  Relative yaw angle : simulink/Logic and Bit Operations/Compare To Constant  relop=>  const=60  OutDataTypeStr=boolean
  Velocity : simulink/Logic and Bit Operations/Compare To Constant  relop=<  const=0.5  OutDataTypeStr=boolean
  Velocity1 : simulink/Logic and Bit Operations/Compare To Constant  relop=<  const=10  OutDataTypeStr=boolean
  isDone : Outport  VectorParamsAs1DForOutWhenUnconnected=off
  wires:
  Velocity/1 -> Logical Operator/1
  Logical Operator/1 -> isDone/1
  v_ego/1 -> Velocity1/1, Velocity/1
  Abs/1 -> Lateral deviation/1
  Lateral deviation/1 -> Logical Operator/2
  e1/1 -> Abs/1
  Velocity1/1 -> AND/1
  e2/1 -> Abs1/1
  Abs1/1 -> R2D/1
  R2D/1 -> Relative yaw angle/1
  Relative yaw angle/1 -> AND/2
  AND/1 -> Logical Operator/3

== system rewardLibrary/Obs // Reward 2-1/Subsystem ==
  v_ego : Inport
  v_ref : Inport  Port=2
  e1 : Inport  Port=3
  e2 : Inport  Port=4
  e1dot : Inport  Port=5
  e2dot : Inport  Port=6
  Add : Sum  Inputs=+-
  Discrete-Time Integrator1 : DiscreteIntegrator  SampleTime=-1  ICPrevOutput=DiscIntNeverNeededParam  ICPrevScaledInput=DiscIntNeverNeededParam
  Discrete-Time Integrator2 : DiscreteIntegrator  SampleTime=-1  ICPrevOutput=DiscIntNeverNeededParam  ICPrevScaledInput=DiscIntNeverNeededParam
  Discrete-Time Integrator3 : DiscreteIntegrator  SampleTime=-1  ICPrevOutput=DiscIntNeverNeededParam  ICPrevScaledInput=DiscIntNeverNeededParam
  Lateral deviation : Scope
  Mux : Mux  Inputs=9
  obs : Outport  VectorParamsAs1DForOutWhenUnconnected=off
  v_err : Outport  Port=2  VectorParamsAs1DForOutWhenUnconnected=off
  wires:
  Add/1 -> v_err/1, Mux/2, Discrete-Time Integrator1/1
  Discrete-Time Integrator3/1 -> Mux/6  "integral_error"
  v_ego/1 -> Add/2, Mux/3
  e1/1 -> Lateral deviation/1, Mux/5, Discrete-Time Integrator2/1
  Discrete-Time Integrator1/1 -> Mux/1  "integral_error"
  e2/1 -> Mux/7, Discrete-Time Integrator3/1
  Discrete-Time Integrator2/1 -> Mux/4  "integral_error"
  Mux/1 -> obs/1
  e1dot/1 -> Mux/8
  e2dot/1 -> Mux/9
  v_ref/1 -> Add/1  "d_rel"

== system rewardLibrary/Obs // Reward 2-1/Subsystem1 ==
  steer : Inport
  e1 : Inport  Port=2
  v_err : Inport  Port=3
  accel : Inport  Port=4
  Compare To Constant : simulink/Logic and Bit Operations/Compare To Constant  relop=<  const=1  OutDataTypeStr=boolean
  Compare To Constant1 : simulink/Logic and Bit Operations/Compare To Constant  relop=<  const=0.25  OutDataTypeStr=boolean
  Gain : Gain  Gain=100
  Gain1 : Gain
  Gain2 : Gain  Gain=500
  Gain3 : Gain  Gain=2
  Gain4 : Gain  Gain=1e-3
  Gain6 : Gain  Gain=100
  Gain7 : Gain  Gain=10
  Math Function2 : Math  Operator=square  SignedPower=on
  Square : Math  Operator=square  SignedPower=on
  Square2 : Math  Operator=square  SignedPower=on
  Square5 : Math  Operator=square  SignedPower=on
  Sum : Sum  Inputs=----
  Sum1 : Sum  Inputs=+++
  Unit Delay : UnitDelay  SampleTime=-1  HasFrameUpgradeWarning=on
  Unit Delay1 : UnitDelay  SampleTime=-1  HasFrameUpgradeWarning=on
  reward : Outport  VectorParamsAs1DForOutWhenUnconnected=off
  wires:
  v_err/1 -> Square5/1
  Square/1 -> Compare To Constant1/1, Gain/1
  Sum1/1 -> reward/1
  accel/1 -> Unit Delay1/1
  Gain6/1 -> Sum/4
  Compare To Constant/1 -> Gain1/1
  Math Function2/1 -> Gain6/1
  Gain3/1 -> Sum1/1
  Compare To Constant1/1 -> Gain3/1
  Square2/1 -> Gain2/1
  Gain7/1 -> Sum/3
  Unit Delay1/1 -> Math Function2/1
  Gain1/1 -> Sum1/3
  steer/1 -> Unit Delay/1
  Gain2/1 -> Sum/2
  Sum/1 -> Gain4/1
  Unit Delay/1 -> Square2/1
  Square5/1 -> Compare To Constant/1, Gain7/1
  Gain/1 -> Sum/1
  Gain4/1 -> Sum1/2
  e1/1 -> Square/1

== system rewardLibrary/Obs // Reward 2-1/Subsystem2 ==
  v_ego : Inport
  e1 : Inport  Port=2
  e2 : Inport  Port=3
  AND : Logic  IconShape=distinctive  AllPortsSameDT=off  OutDataTypeStr=boolean
  Abs : Abs  SaturateOnIntegerOverflow=off
  Abs1 : Abs  SaturateOnIntegerOverflow=off
  Lateral deviation : simulink/Logic and Bit Operations/Compare To Constant  relop=>  const=8  OutDataTypeStr=boolean
  Logical Operator : Logic  Operator=OR  Inputs=3  AllPortsSameDT=off  OutDataTypeStr=boolean
  R2D : Gain  Gain=180/pi
  Relative yaw angle : simulink/Logic and Bit Operations/Compare To Constant  relop=>  const=60  OutDataTypeStr=boolean
  Velocity : simulink/Logic and Bit Operations/Compare To Constant  relop=<  const=0.5  OutDataTypeStr=boolean
  Velocity1 : simulink/Logic and Bit Operations/Compare To Constant  relop=<  const=10  OutDataTypeStr=boolean
  isDone : Outport  VectorParamsAs1DForOutWhenUnconnected=off
  wires:
  Velocity/1 -> Logical Operator/1
  Logical Operator/1 -> isDone/1
  v_ego/1 -> Velocity1/1, Velocity/1
  Abs/1 -> Lateral deviation/1
  Lateral deviation/1 -> Logical Operator/2
  e1/1 -> Abs/1
  Velocity1/1 -> AND/1
  e2/1 -> Abs1/1
  Abs1/1 -> R2D/1
  R2D/1 -> Relative yaw angle/1
  Relative yaw angle/1 -> AND/2
  AND/1 -> Logical Operator/3

== system rewardLibrary/Obs // Reward 2-2/Subsystem ==
  v_ego : Inport
  v_ref : Inport  Port=2
  e1 : Inport  Port=3
  e2 : Inport  Port=4
  e1dot : Inport  Port=5
  e2dot : Inport  Port=6
  Add : Sum  Inputs=+-
  Discrete-Time Integrator1 : DiscreteIntegrator  SampleTime=-1  ICPrevOutput=DiscIntNeverNeededParam  ICPrevScaledInput=DiscIntNeverNeededParam
  Discrete-Time Integrator2 : DiscreteIntegrator  SampleTime=-1  ICPrevOutput=DiscIntNeverNeededParam  ICPrevScaledInput=DiscIntNeverNeededParam
  Discrete-Time Integrator3 : DiscreteIntegrator  SampleTime=-1  ICPrevOutput=DiscIntNeverNeededParam  ICPrevScaledInput=DiscIntNeverNeededParam
  Lateral deviation : Scope
  Mux : Mux  Inputs=9
  obs : Outport  VectorParamsAs1DForOutWhenUnconnected=off
  v_err : Outport  Port=2  VectorParamsAs1DForOutWhenUnconnected=off
  wires:
  Add/1 -> v_err/1, Mux/2, Discrete-Time Integrator1/1
  Discrete-Time Integrator3/1 -> Mux/6  "integral_error"
  v_ego/1 -> Add/2, Mux/3
  e1/1 -> Lateral deviation/1, Mux/5, Discrete-Time Integrator2/1
  Discrete-Time Integrator1/1 -> Mux/1  "integral_error"
  e2/1 -> Mux/7, Discrete-Time Integrator3/1
  Discrete-Time Integrator2/1 -> Mux/4  "integral_error"
  Mux/1 -> obs/1
  e1dot/1 -> Mux/8
  e2dot/1 -> Mux/9
  v_ref/1 -> Add/1  "d_rel"

== system rewardLibrary/Obs // Reward 2-2/Subsystem1 ==
  steer : Inport
  e1 : Inport  Port=2
  v_err : Inport  Port=3
  accel : Inport  Port=4
  Compare To Constant : simulink/Logic and Bit Operations/Compare To Constant  relop=<  const=1  OutDataTypeStr=boolean
  Compare To Constant1 : simulink/Logic and Bit Operations/Compare To Constant  relop=<  const=0.25  OutDataTypeStr=boolean
  Digital Clock : DigitalClock  SampleTime=Ts
  Gain : Gain  Gain=100
  Gain1 : Gain
  Gain2 : Gain  Gain=500
  Gain3 : Gain  Gain=2
  Gain4 : Gain  Gain=1e-3
  Gain5 : Gain  Gain=1/10
  Gain6 : Gain  Gain=100
  Gain7 : Gain  Gain=10
  Math Function2 : Math  Operator=square  SignedPower=on
  Square : Math  Operator=square  SignedPower=on
  Square2 : Math  Operator=square  SignedPower=on
  Square5 : Math  Operator=square  SignedPower=on
  Sum : Sum  Inputs=----
  Sum1 : Sum  Inputs=++++
  Unit Delay : UnitDelay  SampleTime=-1  HasFrameUpgradeWarning=on
  Unit Delay1 : UnitDelay  SampleTime=-1  HasFrameUpgradeWarning=on
  reward : Outport  VectorParamsAs1DForOutWhenUnconnected=off
  wires:
  v_err/1 -> Square5/1
  Square/1 -> Compare To Constant1/1, Gain/1
  Sum1/1 -> reward/1
  accel/1 -> Unit Delay1/1
  Gain6/1 -> Sum/4
  Compare To Constant/1 -> Gain1/1
  Math Function2/1 -> Gain6/1
  Gain3/1 -> Sum1/1
  Compare To Constant1/1 -> Gain3/1
  Square2/1 -> Gain2/1
  Gain7/1 -> Sum/3
  Unit Delay1/1 -> Math Function2/1
  Gain1/1 -> Sum1/3
  steer/1 -> Unit Delay/1
  Gain2/1 -> Sum/2
  Sum/1 -> Gain4/1
  Unit Delay/1 -> Square2/1
  Square5/1 -> Compare To Constant/1, Gain7/1
  Gain/1 -> Sum/1
  Gain4/1 -> Sum1/2
  e1/1 -> Square/1
  Digital Clock/1 -> Gain5/1
  Gain5/1 -> Sum1/4

== system rewardLibrary/Obs // Reward 2-2/Subsystem2 ==
  v_ego : Inport
  e1 : Inport  Port=2
  e2 : Inport  Port=3
  AND : Logic  IconShape=distinctive  AllPortsSameDT=off  OutDataTypeStr=boolean
  Abs : Abs  SaturateOnIntegerOverflow=off
  Abs1 : Abs  SaturateOnIntegerOverflow=off
  Lateral deviation : simulink/Logic and Bit Operations/Compare To Constant  relop=>  const=8  OutDataTypeStr=boolean
  Logical Operator : Logic  Operator=OR  Inputs=3  AllPortsSameDT=off  OutDataTypeStr=boolean
  R2D : Gain  Gain=180/pi
  Relative yaw angle : simulink/Logic and Bit Operations/Compare To Constant  relop=>  const=60  OutDataTypeStr=boolean
  Velocity : simulink/Logic and Bit Operations/Compare To Constant  relop=<  const=0.5  OutDataTypeStr=boolean
  Velocity1 : simulink/Logic and Bit Operations/Compare To Constant  relop=<  const=10  OutDataTypeStr=boolean
  isDone : Outport  VectorParamsAs1DForOutWhenUnconnected=off
  wires:
  Velocity/1 -> Logical Operator/1
  Logical Operator/1 -> isDone/1
  v_ego/1 -> Velocity1/1, Velocity/1
  Abs/1 -> Lateral deviation/1
  Lateral deviation/1 -> Logical Operator/2
  e1/1 -> Abs/1
  Velocity1/1 -> AND/1
  e2/1 -> Abs1/1
  Abs1/1 -> R2D/1
  R2D/1 -> Relative yaw angle/1
  Relative yaw angle/1 -> AND/2
  AND/1 -> Logical Operator/3

== system rewardLibrary/Obs // Reward 2-3/Subsystem ==
  v_ego : Inport
  v_ref : Inport  Port=2
  e1 : Inport  Port=3
  e2 : Inport  Port=4
  e1dot : Inport  Port=5
  e2dot : Inport  Port=6
  Add : Sum  Inputs=+-
  Discrete-Time Integrator1 : DiscreteIntegrator  SampleTime=-1  ICPrevOutput=DiscIntNeverNeededParam  ICPrevScaledInput=DiscIntNeverNeededParam
  Discrete-Time Integrator2 : DiscreteIntegrator  SampleTime=-1  ICPrevOutput=DiscIntNeverNeededParam  ICPrevScaledInput=DiscIntNeverNeededParam
  Discrete-Time Integrator3 : DiscreteIntegrator  SampleTime=-1  ICPrevOutput=DiscIntNeverNeededParam  ICPrevScaledInput=DiscIntNeverNeededParam
  Lateral deviation : Scope
  Mux : Mux  Inputs=9
  obs : Outport  VectorParamsAs1DForOutWhenUnconnected=off
  v_err : Outport  Port=2  VectorParamsAs1DForOutWhenUnconnected=off
  wires:
  Add/1 -> v_err/1, Mux/2, Discrete-Time Integrator1/1
  Discrete-Time Integrator3/1 -> Mux/6  "integral_error"
  v_ego/1 -> Add/2, Mux/3
  e1/1 -> Lateral deviation/1, Mux/5, Discrete-Time Integrator2/1
  Discrete-Time Integrator1/1 -> Mux/1  "integral_error"
  e2/1 -> Mux/7, Discrete-Time Integrator3/1
  Discrete-Time Integrator2/1 -> Mux/4  "integral_error"
  Mux/1 -> obs/1
  e1dot/1 -> Mux/8
  e2dot/1 -> Mux/9
  v_ref/1 -> Add/1  "d_rel"

== system rewardLibrary/Obs // Reward 2-3/Subsystem1 ==
  steer : Inport
  e1 : Inport  Port=2
  v_err : Inport  Port=3
  accel : Inport  Port=4
  Compare To Constant : simulink/Logic and Bit Operations/Compare To Constant  relop=<  const=1  OutDataTypeStr=boolean
  Compare To Constant1 : simulink/Logic and Bit Operations/Compare To Constant  relop=<  const=4  OutDataTypeStr=boolean
  Digital Clock : DigitalClock  SampleTime=Ts
  Gain : Gain  Gain=100
  Gain1 : Gain
  Gain2 : Gain  Gain=500
  Gain3 : Gain  Gain=2
  Gain4 : Gain  Gain=1e-3
  Gain5 : Gain  Gain=1/10
  Gain6 : Gain  Gain=100
  Gain7 : Gain  Gain=10
  Math Function2 : Math  Operator=square  SignedPower=on
  Square : Math  Operator=square  SignedPower=on
  Square2 : Math  Operator=square  SignedPower=on
  Square5 : Math  Operator=square  SignedPower=on
  Sum : Sum  Inputs=----
  Sum1 : Sum  Inputs=++++
  Unit Delay : UnitDelay  SampleTime=-1  HasFrameUpgradeWarning=on
  Unit Delay1 : UnitDelay  SampleTime=-1  HasFrameUpgradeWarning=on
  reward : Outport  VectorParamsAs1DForOutWhenUnconnected=off
  wires:
  v_err/1 -> Square5/1
  Square/1 -> Compare To Constant1/1, Gain/1
  Sum1/1 -> reward/1
  accel/1 -> Unit Delay1/1
  Gain6/1 -> Sum/4
  Compare To Constant/1 -> Gain1/1
  Math Function2/1 -> Gain6/1
  Gain3/1 -> Sum1/1
  Compare To Constant1/1 -> Gain3/1
  Square2/1 -> Gain2/1
  Gain7/1 -> Sum/3
  Unit Delay1/1 -> Math Function2/1
  Gain1/1 -> Sum1/3
  steer/1 -> Unit Delay/1
  Gain2/1 -> Sum/2
  Sum/1 -> Gain4/1
  Unit Delay/1 -> Square2/1
  Square5/1 -> Compare To Constant/1, Gain7/1
  Gain/1 -> Sum/1
  Gain4/1 -> Sum1/2
  e1/1 -> Square/1
  Digital Clock/1 -> Gain5/1
  Gain5/1 -> Sum1/4
